simulink model "crossproduct_test"  (Simulink 8.4)
settings: Solver=VariableStepDiscrete  StartTime=0.0  StopTime=0  MaxStep=1  RelTol=1e-3
libraries: vrlib x2
settings Model: Creator=arnaud  LastModifiedBy=arnaud
settings DataIOCC: ExternalInput=xin  SaveFormat=Structure

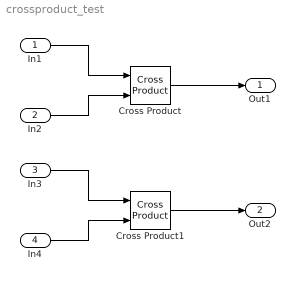
== system crossproduct_test ==
  In1 : Inport  PortDimensions=3
      settings: SignalType=complex
  In2 : Inport  Port=2  PortDimensions=3
  In3 : Inport  Port=3  PortDimensions=3
  In4 : Inport  Port=4  PortDimensions=3
  Cross Product : vrlib/Utilities/Cross Product
  Cross Product1 : vrlib/Utilities/Cross Product
  Out1 : Outport
  Out2 : Outport  Port=2
  wires:
  Cross Product/1 -> Out1/1
  In1/1 -> Cross Product/1
  In2/1 -> Cross Product/2
  Cross Product1/1 -> Out2/1
  In3/1 -> Cross Product1/1
  In4/1 -> Cross Product1/2
